simulink model "LinProgTest"  (R2017a)
settings: Solver=VariableStepAuto  StartTime=0.0  StopTime=10.0  RelTol=1e-3
settings Model: Creator=erich  LastModifiedBy=erich

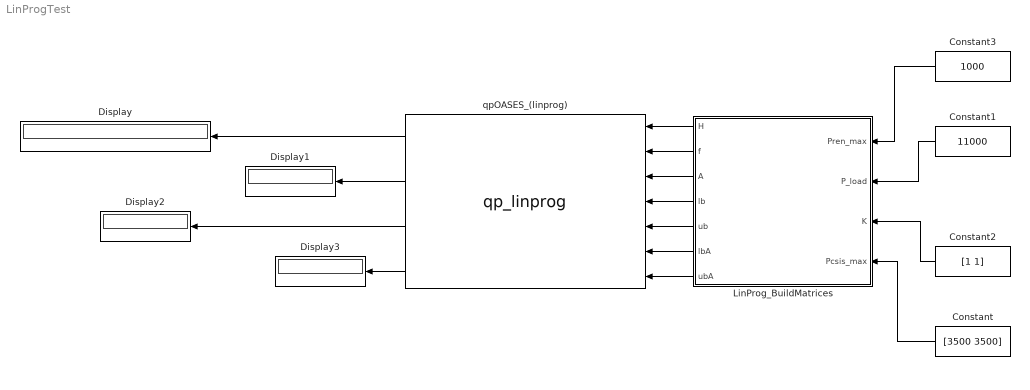
== system LinProgTest ==
  Constant : Constant  Value=[3500 3500]
  Constant1 : Constant  Value=11000
  Constant2 : Constant  Value=[1 1]
  Constant3 : Constant  Value=1000
  Display{,1..3} (4 alike) : Display
  LinProg_BuildMatrices : MATLAB Function  TreatAsAtomicUnit=on
  qpOASES_(linprog) : S-Function  FunctionName=qp_linprog  SFunctionDeploymentMode=off  EnableBusSupport=off
  wires:
  LinProg_BuildMatrices/5(ub) -> qpOASES_(linprog)/5
  LinProg_BuildMatrices/2(f) -> qpOASES_(linprog)/2
  LinProg_BuildMatrices/3(A) -> qpOASES_(linprog)/3
  LinProg_BuildMatrices/6(lbA) -> qpOASES_(linprog)/6
  LinProg_BuildMatrices/7(ubA) -> qpOASES_(linprog)/7
  LinProg_BuildMatrices/4(lb) -> qpOASES_(linprog)/4
  LinProg_BuildMatrices/1(H) -> qpOASES_(linprog)/1
  qpOASES_(linprog)/1 -> Display/1
  qpOASES_(linprog)/2 -> Display1/1
  qpOASES_(linprog)/3 -> Display2/1
  qpOASES_(linprog)/4 -> Display3/1
  Constant1/1 -> LinProg_BuildMatrices/2(P_load)
  Constant2/1 -> LinProg_BuildMatrices/3(K)
  Constant3/1 -> LinProg_BuildMatrices/1(Pren_max)
  Constant/1 -> LinProg_BuildMatrices/4(Pcsis_max)

== matlab function LinProgTest/LinProg_BuildMatrices ==
  data: H output; Pren_max input; f output; P_load input; K input; A output; lb output; ub output; lbA output; ubA output; Pcsis_max input
function [H, f, A, lb, ub, lbA, ubA] = fcn(Pren_max, P_load, K, Pcsis_max)

% Pr_max es la potencia maxima que puede suministrar el nodo de energias
% renovables.

% P_load es la potencia que consume la carga. ambas potencias son un vector
% de 2 componentes donde la primera componenete es la potencia activa y la
% segunda componenete es la potencia reactiva.

% Kp y Kq corresponde a un vector con los costos de la energia activa y 
% reactiva respectivamente para cada uno de los convertidores, en este caso
% bio y diesel solamente pero pueden agregarse tantas fuentes como se
% desee.

% Pin_max Qin_max corresponde a un vector con los valores maximos de
% potencia activa y reactiva que pueden generar cada una de las otras 
% fuentes diferentes a energias alternativas.


% El bloque qpOASES_(linprog) es un bloque que resuelve el problema standar
% de optimizacion cuadratica :
% 1/2 x' H x + x' f
% sujeto a unas restricciones. la matriz H corresponde a la parte
% cuadratica del problema mientras que f corresponde a la parte lineal. es
% decir que haciendo H = matriz de zeros, es posible reutilizar el bloque
% para solucionar problemas de programacion lineal, que es justamente lo
% que se hace en esta parte del modelo.

% La presente matlab function tiene como tarea formar las matrices f
% y A de restricciones apropiadas para que el bloque de qp oases realice la
% funcione de programacion lineal.

Pm = sum(Pcsis_max); % potencia activa maxima que pueden entregar todas las fuentes (en este caso bio y diesel)


D = P_load - Pren_max; % diferencia entre la potencia que puede generar
% renovables con la que consume la carga.


     % % % % % % % % % % % % % % % % % % % % % % % % % % % % %  
    % Formacion de las entradas para la programacion lineal.  %
     % % % % % % % % % % % % % % % % % % % % % % % % % % % % %  
     
% parte cuadratica de la funcion de coste que se pone en zeros para
% transformarlo en un problema de programacion lineal.
H = zeros(1, length(K)^2);

% funcion de coste lineal.
f = K;

% matriz de restricciones.
% esta formada con la idea de definir que la suma de todas las potencias
% deben almenos cubrir la cantidad de energia activa y reactiva que no
% puede suministrar renovables.
A = ones(1, length(K));

lb = zeros(1, length(K)); % potencia minima que puede generar cada uno de los generadores.
ub = [Pcsis_max]; % potencia maxima que pueden generar cada uno de los generadores.

ubA = [Pm]; % tambien esta relacionado con la potencia min, es un
% requerimiento para el blque de programacion lineal.

% depenediendo la diferencia entre la potencia que pide la carga y la que
% pueden suministrar energias renovables entonces lbA debe establecerce de
% manera conveniente para que el problema de programacion lineal tenga
% solucion.

% restriccion limite inferior para la potencia activa
if(D > 0) % en caso de que renovables no baste para alimentar la carga...
    if(D >= Pm)
        vp = Pm;
    else
        vp = D(1);
    end
else % si renovables basta para alimentar la carga. es decir D = 0 ó negativo
    vp = 0;
end

lbA = vp;
